simulink model "dpf_warning_shell"  (R2019a)
settings: Solver=VariableStepAuto  StartTime=0.0  StopTime=10.0  RelTol=1e-3
settings Model: DataDictionary=out7.sldd  Creator=admin  LastModifiedBy=User

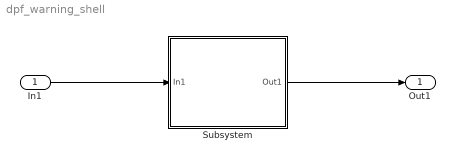
== system dpf_warning_shell ==
  In1 : Inport
  Subsystem : Subsystem
  Out1 : Outport
  wires:
  In1/1 -> Subsystem/1(In1)
  Subsystem/1(Out1) -> Out1/1

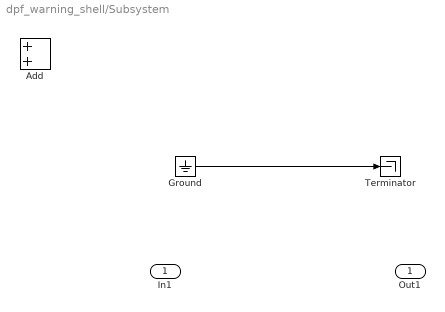
== system dpf_warning_shell/Subsystem ==
  In1 : Inport
  Add : Sum
  Ground : Ground
  Terminator : Terminator
  Out1 : Outport
  wires:
  Ground/1 -> Terminator/1
